simulink library "netZeroSpoolingController_ul"  (R2020a)
settings: Solver=VariableStepAuto  StartTime=0.0  StopTime=10.0  RelTol=1e-3
undefined symbols (not defined in the file or in its folder): fltCtrl, SPOOLINGCONTROLLER
libraries: simulink x8, runningAvg_ul x2, dspsigops x1, filteredPIDController_ul x1, stopwatch_ul x1
settings Model: Creator=James Reed  LastModifiedBy=Josh Gaming
settings DataIOCC: ReturnWorkspaceOutputs=off
settings DebuggingCC: ArithmeticOperatorsInVariantConditions=warning
settings SFSimCC: CustomCodeUndefinedFunction=UseInterfaceOnly

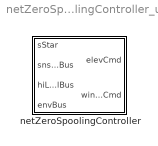
== system netZeroSpoolingController_ul ==
  netZeroSpoolingController : Subsystem  VariantControl=strcmpi(SPOOLINGCONTROLLER,'netZeroSpoolingController')  mask{reelInDefl=fltCtrl.elevatorReelInDef.Value, reelOutDefl=0, sigmaVecInit=[0.25 0.125], firstSpoolLap=fltCtrl.firstSpoolLap.Value}
      mask prompts: reelInDefl "Reel In Elevator Deflection [deg]"; reelOutDefl "Reel Out Elevator Deflection [deg]"; sigmaVecInit "Init Spooling Param Vec [center width]"; firstSpoolLap "First Lap to Begin Spooling"
      mask TypeOptions reelInDefl: ReelInElevDefl1/Value
      mask TypeOptions reelOutDefl: ReelOutElevDefl1/Value

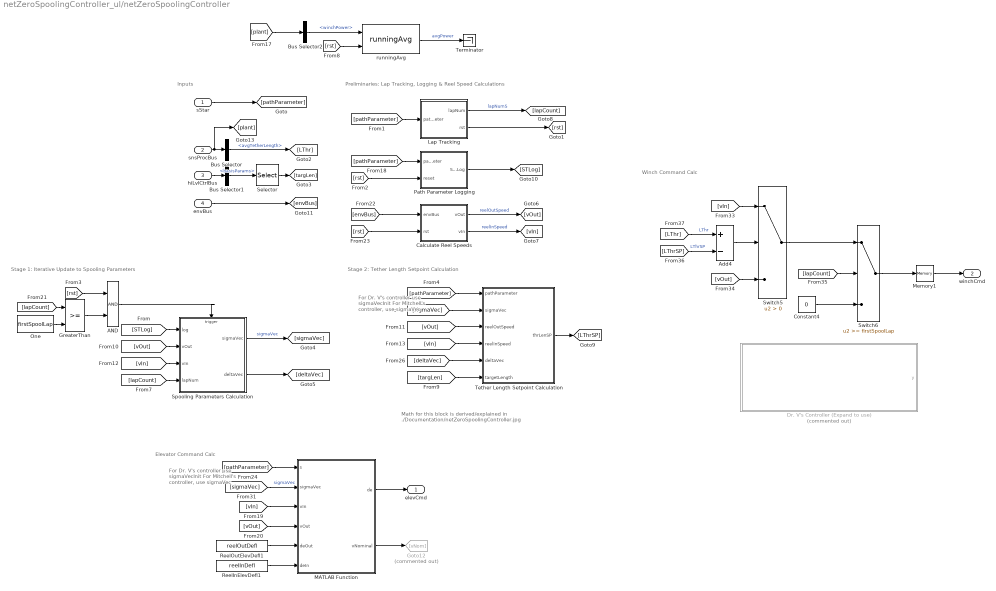
== system netZeroSpoolingController_ul/netZeroSpoolingController ==
  note: Elevator Command Calc
  note: Winch Command Calc
  note: For Dr. V's controller use sigmaVecInit
      |
      | For Mitchell's controller, use sigmaVec
  note: Math for this block is derived/explained in
      | ./Documentation/netZeroSpoolingController.jpg
  note: Stage 1: Iterative Update to Spooling Parameters
  note: Stage 2: Tether Length Setpoint Calculation
  note: Inputs
  note: Preliminaries: Lap Tracking, Logging & Reel Speed Calculations
  note: For Dr. V's controller use sigmaVecInit
      |
      | For Mitchell's controller, use sigmaVec
  "sStar " : Inport
  snsProcBus : Inport  Port=2  OutDataTypeStr=Bus: sensorsProcessingBus
  hiLvlCtrlBus : Inport  Port=3  OutDataTypeStr=Bus: hiLvlCtrlBus
  envBus : Inport  Port=4  OutDataTypeStr=Bus: envBus
  AND : Logic  AllPortsSameDT=off  OutDataTypeStr=boolean
  Add4 : Sum  Inputs=+-
  Bus Selector : BusSelector  OutputSignals=avgTetherLength
  Bus Selector1 : BusSelector  OutputSignals=basisParams
  Bus Selector2 : BusSelector  OutputSignals=winchPower
  Calculate Reel Speeds : Subsystem
  Constant4 : Constant  Value=0
  Dr. V's Controller (Expand to use) : Subsystem  Commented=on
  Goto12 : Goto  Commented=on  GotoTag=vNom
  GreaterThan : RelationalOperator  OutDataTypeStr=boolean  RndMeth=Simplest
  Lap Tracking : Subsystem
  MATLAB Function : MATLAB Function  TreatAsAtomicUnit=on
  Memory1 : Memory
  One : Constant  Value=firstSpoolLap  OutDataTypeStr=Inherit: Inherit via back propagation
  Path Parameter Logging : Subsystem
  ReelInElevDefl1 : Constant  Value=reelInDefl
  ReelOutElevDefl1 : Constant  Value=reelOutDefl
  Selector : Selector  InputPortWidth=5  IndexOptions=Index vector (dialog)  Indices=5  OutputSizes=1
  Spooling Parameters Calculation : Subsystem  TreatAsAtomicUnit=on
  Switch5 : Switch  Criteria=u2 > Threshold
  Switch6 : Switch  Threshold=firstSpoolLap
  Terminator : Terminator
  Tether Length Setpoint Calculation : Subsystem
  runningAvg : runningAvg_ul/runningAvg  SystemSampleTime=-1  Latency=0  AutoFrameSizeCalculation=off
  elevCmd : Outport  VectorParamsAs1DForOutWhenUnconnected=off
  "winchCmd " : Outport  Port=2  VectorParamsAs1DForOutWhenUnconnected=off
  wires:
  AND/1 -> Spooling Parameters Calculation/Trigger
  GreaterThan/1 -> AND/2
  [rst] -> AND/1
  One/1 -> GreaterThan/2
  [lapCount] -> GreaterThan/1
  hiLvlCtrlBus/1 -> Bus Selector1/1
  "sStar "/1 -> [pathParameter]
  Bus Selector/1 -> [LThr]  "<avgTetherLength>"
  Spooling Parameters Calculation/1(sigmaVec) -> [sigmaVec]  "sigmaVec"
  Spooling Parameters Calculation/2(deltaVec) -> [deltaVec]
  [vOut] -> Spooling Parameters Calculation/2(vOut)
  [vIn] -> Spooling Parameters Calculation/3(vIn)
  [pathParameter] -> Path Parameter Logging/1(pathParameter)
  [rst] -> Path Parameter Logging/2(reset)
  Path Parameter Logging/1(SVsTLog) -> [STLog]
  [STLog] -> Spooling Parameters Calculation/1(log)
  envBus/1 -> [envBus]
  [envBus] -> Calculate Reel Speeds/1(envBus)
  Calculate Reel Speeds/1(vOut) -> [vOut]  "reelOutSpeed"
  Calculate Reel Speeds/2(vIn) -> [vIn]  "reelInSpeed"
  [rst] -> Calculate Reel Speeds/2(rst)
  [pathParameter] -> Lap Tracking/1(pathParameter)
  Lap Tracking/1(lapNum) -> [lapCount]  "lapNumS"
  Lap Tracking/2(rst) -> [rst]
  [pathParameter] -> Tether Length Setpoint Calculation/1(pathParameter)
  [sigmaVec] -> Tether Length Setpoint Calculation/2(sigmaVec)
  [vOut] -> Tether Length Setpoint Calculation/3(reelOutSpeed)
  [vIn] -> Tether Length Setpoint Calculation/4(reelInSpeed)
  [deltaVec] -> Tether Length Setpoint Calculation/5(deltaVec)
  Tether Length Setpoint Calculation/1(thrLenSP) -> [LThrSP]
  [lapCount] -> Spooling Parameters Calculation/4(lapNum)
  Bus Selector1/1 -> Selector/1  "<basisParams>"
  Selector/1 -> [targLen]
  [targLen] -> Tether Length Setpoint Calculation/6(targetLength)
  [pathParameter] -> MATLAB Function/1(s)
  [vIn] -> MATLAB Function/3(vIn)
  [vOut] -> MATLAB Function/4(vOut)
  ReelInElevDefl1/1 -> MATLAB Function/6(deIn)
  ReelOutElevDefl1/1 -> MATLAB Function/5(deOut)
  MATLAB Function/1(de) -> elevCmd/1
  MATLAB Function/2(vNominal) -> Goto12/1
  [lapCount] -> Switch6/2
  Constant4/1 -> Switch6/3
  [LThrSP] -> Add4/2  "LThrSP"
  Add4/1 -> Switch5/2
  [vOut] -> Switch5/3
  Switch5/1 -> Switch6/1
  [vIn] -> Switch5/1
  [LThr] -> Add4/1  "LThr"
  [rst] -> runningAvg/2
  Bus Selector2/1 -> runningAvg/1  "<winchPower>"
  runningAvg/1 -> Terminator/1  "avgPower"
  snsProcBus/1 -> [plant], Bus Selector/1
  [plant] -> Bus Selector2/1
  [sigmaVec] -> MATLAB Function/2(sigmaVec)  "sigmaVec"
  Switch6/1 -> Memory1/1
  Memory1/1 -> "winchCmd "/1

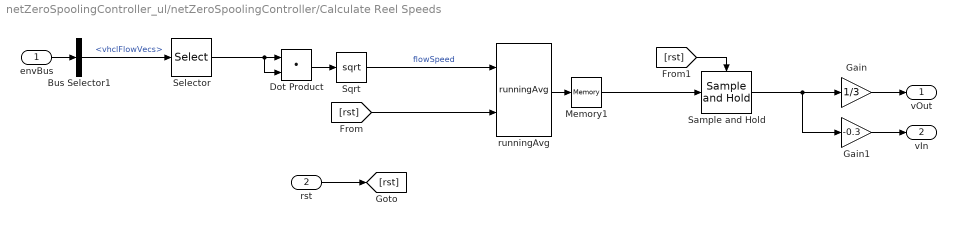
== system netZeroSpoolingController_ul/netZeroSpoolingController/Calculate Reel Speeds ==
  envBus : Inport
  rst : Inport  Port=2
  Bus Selector1 : BusSelector  OutputSignals=vhclFlowVecs
  Dot Product : DotProduct  InputSameDT=on  OutDataTypeStr=Inherit: Inherit via internal rule
  Gain : Gain  Gain=1/3
  Gain1 : Gain  Gain=-0.3
  Memory1 : Memory
  Sample and Hold : dspsigops/Sample and Hold  trig=Rising edge  initCond=0  latchinput=off
  Selector : Selector  NumberOfDimensions=2  InputPortWidth=3  IndexOptions=Select all,Index vector (dialog)  Indices=[1 3],5  OutputSizes=1,1
  Sqrt : Sqrt  SaturateOnIntegerOverflow=on
  runningAvg : runningAvg_ul/runningAvg  SystemSampleTime=-1  Latency=0  AutoFrameSizeCalculation=off
  vOut : Outport  VectorParamsAs1DForOutWhenUnconnected=off
  vIn : Outport  Port=2  VectorParamsAs1DForOutWhenUnconnected=off
  wires:
  Gain1/1 -> vIn/1
  Gain/1 -> vOut/1
  Sample and Hold/1 -> Gain1/1, Gain/1
  rst/1 -> [rst]
  Bus Selector1/1 -> Selector/1  "<vhclFlowVecs>"
  runningAvg/1 -> Memory1/1
  Sqrt/1 -> runningAvg/1  "flowSpeed"
  envBus/1 -> Bus Selector1/1
  Memory1/1 -> Sample and Hold/1
  [rst] -> runningAvg/2
  [rst] -> Sample and Hold/Trigger
  Selector/1 -> Dot Product/2, Dot Product/1
  Dot Product/1 -> Sqrt/1

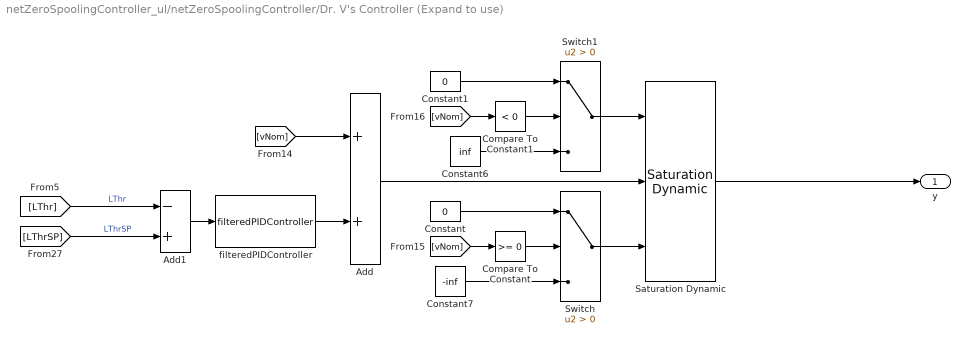
== system netZeroSpoolingController_ul/netZeroSpoolingController/Dr. V's Controller (Expand to use) ==
  Add : Sum
  Add1 : Sum  Inputs=-+
  Compare To Constant : simulink/Logic and Bit Operations/Compare To Constant  relop=>=  const=0  OutDataTypeStr=boolean
  Compare To Constant1 : simulink/Logic and Bit Operations/Compare To Constant  relop=<  const=0  OutDataTypeStr=boolean
  Constant : Constant  Value=0
  Constant1 : Constant  Value=0
  Constant6 : Constant  Value=inf
  Constant7 : Constant  Value=-inf
  Saturation Dynamic : simulink/Discontinuities/Saturation Dynamic  OutMin=[]  OutMax=[]  OutDataTypeStr=Inherit: Same as second input  OutDataType=fixdt(1, 16)  OutScaling=2^-10  DoSatur=off
  Switch : Switch  Criteria=u2 > Threshold
  Switch1 : Switch  Criteria=u2 > Threshold
  filteredPIDController : filteredPIDController_ul/filteredPIDController  kp=.1  ki=0  kd=0  Value=0  externalReset=none
  y : Outport
  wires:
  Compare To Constant1/1 -> Switch1/2
  Add/1 -> Saturation Dynamic/2
  [LThrSP] -> Add1/2  "LThrSP"
  [vNom] -> Compare To Constant/1
  Compare To Constant/1 -> Switch/2
  Add1/1 -> filteredPIDController/1
  Switch/1 -> Saturation Dynamic/3
  Constant6/1 -> Switch1/3
  filteredPIDController/1 -> Add/2
  Switch1/1 -> Saturation Dynamic/1
  [vNom] -> Compare To Constant1/1
  Constant/1 -> Switch/1
  [vNom] -> Add/1
  Constant1/1 -> Switch1/1
  [LThr] -> Add1/1  "LThr"
  Constant7/1 -> Switch/3
  Saturation Dynamic/1 -> y/1

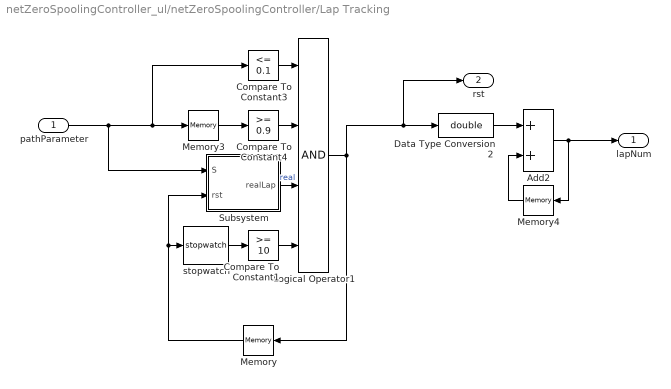
== system netZeroSpoolingController_ul/netZeroSpoolingController/Lap Tracking ==
  pathParameter : Inport
  Add2 : Sum
  Compare To Constant1 : simulink/Logic and Bit Operations/Compare To Constant  relop=>=  const=10  OutDataTypeStr=boolean
  Compare To Constant3 : simulink/Logic and Bit Operations/Compare To Constant  relop=<=  const=0.1  OutDataTypeStr=boolean
  Compare To Constant4 : simulink/Logic and Bit Operations/Compare To Constant  relop=>=  const=0.9  OutDataTypeStr=boolean
  Data Type Conversion2 : DataTypeConversion  OutDataTypeStr=double
  Logical Operator1 : Logic  Inputs=4  AllPortsSameDT=off  OutDataTypeStr=boolean
  Memory : Memory  InitialCondition=false
  Memory3 : Memory
  Memory4 : Memory
  Subsystem : Subsystem
  stopwatch : stopwatch_ul/stopwatch  SystemSampleTime=-1  Latency=0  AutoFrameSizeCalculation=off
  lapNum : Outport  VectorParamsAs1DForOutWhenUnconnected=off
  rst : Outport  Port=2  VectorParamsAs1DForOutWhenUnconnected=off
  wires:
  Compare To Constant3/1 -> Logical Operator1/1
  Memory3/1 -> Compare To Constant4/1
  Data Type Conversion2/1 -> Add2/1
  Logical Operator1/1 -> rst/1, Data Type Conversion2/1, Memory/1
  Memory4/1 -> Add2/2
  Add2/1 -> lapNum/1, Memory4/1
  Compare To Constant4/1 -> Logical Operator1/2
  pathParameter/1 -> Subsystem/1(S), Compare To Constant3/1, Memory3/1
  stopwatch/1 -> Compare To Constant1/1
  Memory/1 -> Subsystem/2(rst), stopwatch/1
  Compare To Constant1/1 -> Logical Operator1/4
  Subsystem/1(realLap) -> Logical Operator1/3  "real"

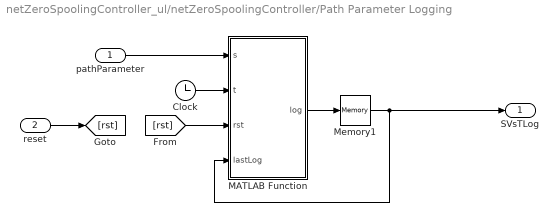
== system netZeroSpoolingController_ul/netZeroSpoolingController/Path Parameter Logging ==
  pathParameter : Inport
  reset : Inport  Port=2
  Clock : Clock
  MATLAB Function : MATLAB Function  TreatAsAtomicUnit=on
  Memory1 : Memory  InitialCondition=zeros(1000,2)
  SVsTLog : Outport  VectorParamsAs1DForOutWhenUnconnected=off
  wires:
  MATLAB Function/1(log) -> Memory1/1
  reset/1 -> [rst]
  pathParameter/1 -> MATLAB Function/1(s)
  Clock/1 -> MATLAB Function/2(t)
  Memory1/1 -> SVsTLog/1, MATLAB Function/4(lastLog)
  [rst] -> MATLAB Function/3(rst)

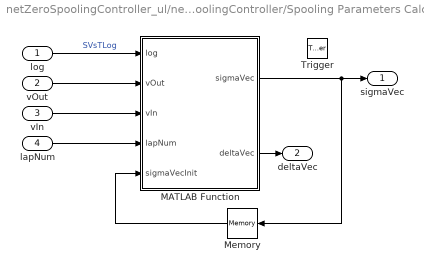
== system netZeroSpoolingController_ul/netZeroSpoolingController/Spooling Parameters Calculation ==
  log : Inport
  vOut : Inport  Port=2
  vIn : Inport  Port=3
  lapNum : Inport  Port=4
  Trigger : TriggerPort  VariantControl=Variant
  MATLAB Function : MATLAB Function  TreatAsAtomicUnit=on
  Memory : Memory  InitialCondition=sigmaVecInit  InheritSampleTime=on
  sigmaVec : Outport  InitialOutput=sigmaVecInit  VectorParamsAs1DForOutWhenUnconnected=off
  deltaVec : Outport  Port=2  InitialOutput="[0.0136    0.0097    0.0198    0.0152    0.0208]"  VectorParamsAs1DForOutWhenUnconnected=off
  wires:
  log/1 -> MATLAB Function/1(log)  "SVsTLog"
  Memory/1 -> MATLAB Function/5(sigmaVecInit)
  vOut/1 -> MATLAB Function/2(vOut)
  vIn/1 -> MATLAB Function/3(vIn)
  MATLAB Function/2(deltaVec) -> deltaVec/1
  MATLAB Function/1(sigmaVec) -> Memory/1, sigmaVec/1
  lapNum/1 -> MATLAB Function/4(lapNum)

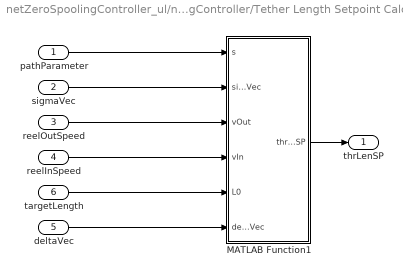
== system netZeroSpoolingController_ul/netZeroSpoolingController/Tether Length Setpoint Calculation ==
  pathParameter : Inport
  sigmaVec : Inport  Port=2
  reelOutSpeed : Inport  Port=3
  reelInSpeed : Inport  Port=4
  deltaVec : Inport  Port=5
  targetLength : Inport  Port=6
  MATLAB Function1 : MATLAB Function  TreatAsAtomicUnit=on
  thrLenSP : Outport  VectorParamsAs1DForOutWhenUnconnected=off
  wires:
  sigmaVec/1 -> MATLAB Function1/2(sigmaVec)
  reelInSpeed/1 -> MATLAB Function1/4(vIn)
  reelOutSpeed/1 -> MATLAB Function1/3(vOut)
  pathParameter/1 -> MATLAB Function1/1(s)
  MATLAB Function1/1(thrLenSP) -> thrLenSP/1
  deltaVec/1 -> MATLAB Function1/6(deltaVec)
  targetLength/1 -> MATLAB Function1/5(L0)

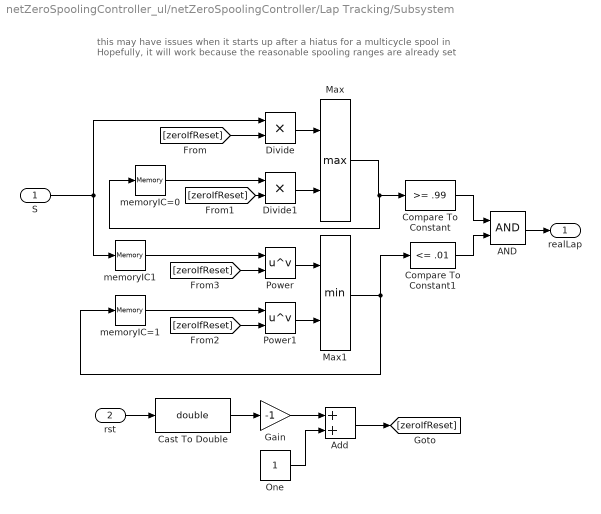
== system netZeroSpoolingController_ul/netZeroSpoolingController/Lap Tracking/Subsystem ==
  note: this may have issues when it starts up after a hiatus for a multicycle spool in
      | Hopefully, it will work because the reasonable spooling ranges are already set
  S : Inport
  rst : Inport  Port=2
  AND : Logic  AllPortsSameDT=off  OutDataTypeStr=boolean
  Add : Sum
  Cast To Double : DataTypeConversion  OutDataTypeStr=double
  Compare To Constant : simulink/Logic and Bit Operations/Compare To Constant  relop=>=  const=.99  OutDataTypeStr=boolean
  Compare To Constant1 : simulink/Logic and Bit Operations/Compare To Constant  relop=<=  const=.01  OutDataTypeStr=boolean
  Divide : Product  Inputs=**
  Divide1 : Product  Inputs=**
  Gain : Gain  Gain=-1
  Max : MinMax  Function=max  Inputs=2
  Max1 : MinMax  Inputs=2
  One : Constant  OutDataTypeStr=Inherit: Inherit via back propagation
  Power : Math  Operator=pow  SaturateOnIntegerOverflow=on
  Power1 : Math  Operator=pow  SaturateOnIntegerOverflow=on
  memoryIC1 : Memory  InitialCondition=1
  memoryIC=0 : Memory
  memoryIC=1 : Memory  InitialCondition=1
  realLap : Outport
  wires:
  Max1/1 -> Compare To Constant1/1, memoryIC=1/1
  rst/1 -> Cast To Double/1
  S/1 -> Divide/1, memoryIC1/1
  Gain/1 -> Add/1
  Add/1 -> [zeroIfReset]
  One/1 -> Add/2
  Divide/1 -> Max/1
  Max/1 -> memoryIC=0/1, Compare To Constant/1
  Power/1 -> Max1/1
  Power1/1 -> Max1/2
  Cast To Double/1 -> Gain/1
  Compare To Constant/1 -> AND/1
  Compare To Constant1/1 -> AND/2
  AND/1 -> realLap/1
  [zeroIfReset] -> Divide/2
  [zeroIfReset] -> Power/2
  [zeroIfReset] -> Divide1/2
  Divide1/1 -> Max/2
  memoryIC=0/1 -> Divide1/1
  [zeroIfReset] -> Power1/2
  memoryIC=1/1 -> Power1/1
  memoryIC1/1 -> Power/1

== matlab function netZeroSpoolingController_ul/netZeroSpoolingController/Spooling Parameters Calculation/MATLAB Function ==
  data: log input; vOut input; vIn input; lapNum input; sigmaVecInit input; sigmaVec output; deltaVec output
function [sigmaVec,deltaVec] = fcn(log,vOut,vIn,lapNum,sigmaVecInit)

sc = sigmaVecInit(1);
sw = sigmaVecInit(2);
sigmaVec = sigmaVecInit;

cleanLog = [0 0;...
    log(and(log(:,1)~=0,log(:,2)~=0),:)];
 
% Extract regions
r1 = cleanLog(and(cleanLog(:,1)>=0        ,cleanLog(:,1)<sc-sw),:);
r2 = cleanLog(and(cleanLog(:,1)>=sc-sw    ,cleanLog(:,1)<sc+sw),:);
r3 = cleanLog(and(cleanLog(:,1)>=sc+sw    ,cleanLog(:,1)<0.5+sc-sw),:);
r4 = cleanLog(and(cleanLog(:,1)>=0.5+sc-sw,cleanLog(:,1)<0.5+sc+sw),:);
r5 = cleanLog(and(cleanLog(:,1)>=0.5+sc+sw,cleanLog(:,1)<=1),:);

% Calculate average numerical derivative in each region ds/dt
ds1 = mean(diff(r1(:,1))./diff(r1(:,2)));
ds2 = mean(diff(r2(:,1))./diff(r2(:,2)));
ds3 = mean(diff(r3(:,1))./diff(r3(:,2)));
ds4 = mean(diff(r4(:,1))./diff(r4(:,2)));
ds5 = mean(diff(r5(:,1))./diff(r5(:,2)));

deltaVec = [ds1 ds2 ds3 ds4 ds5]';

dsInv = diag([1/ds1 1/ds2 1/ds3 1/ds4 1/ds5]);

V = diag([vOut vIn vOut vIn vOut]);

Delta = eye(5);
Delta(2,1) = -1;
Delta(3,2) = -1;
Delta(4,3) = -1;
Delta(5,4) = -1;

A  = [ 0  0 0.5 0.5 1]';
B1 = [ 1  1   1   1 0]';
B2 = [-1  1  -1   1 0]';

c1 = ones(1,5)*V*dsInv*Delta*(A+B1*sc);
c2 = ones(1,5)*V*dsInv*Delta*B2;
sw = min([max([-c1/c2 0]) sc]); % 0<=sw<=sc
sigmaVec(2) = sw;

% Note: the following code alternates between updating sc and sw.
% After a bit of testing, I found that the update on sc was really screwing
% things up.  Not sure why that is at the moment, but it's kind of
% irrelevant since the update on sw alone works well enough.  Moving on.
% -MC

% Alternate updaing sc and sw each lap
% if mod(round(lapNum),2) % Odd lap number
    % Case 1, sc fixed, update sw
%     sigmaVec(1) = sc;
%     c1 = ones(1,5)*V*dsInv*Delta*(A+B1*sc);
%     c2 = ones(1,5)*V*dsInv*Delta*B2;
%     sw = min([max([-c1/c2 0]) sc]); % 0<=sw<=0.25
% else % Even lap number
%     % Case 2, sw fixed, update sc
% %     sigmaVec(2) = sw;
%     c1 = ones(1,5)*V*dsInv*Delta*(A+B2*sw);
%     c2 = ones(1,5)*V*dsInv*Delta*B1;
%     sc = min([max([-c1/c2 sw]) 0.5-sw]);
% end

% sigmaVec(1) = sc;
% sigmaVec(2) = sw;

== matlab function netZeroSpoolingController_ul/netZeroSpoolingController/Path Parameter Logging/MATLAB Function ==
  data: s input; log output; t input; rst input; lastLog input
function log = fcn(s,t,rst,lastLog)
% function that logs the path position and time into a matrix
% [pathPosition,t]
if rst
    lastLog = nan(1000,2);
end
log = lastLog;
idx = min([max([round(s*1000),1]),1000]);
log(idx,1) = s;
log(idx,2) = t;

== matlab function netZeroSpoolingController_ul/netZeroSpoolingController/Tether Length Setpoint Calculation/MATLAB Function1 ==
  data: s input; thrLenSP output; sigmaVec input; vOut input; vIn input; L0 input; deltaVec input
function thrLenSP  = fcn(s,sigmaVec,vOut,vIn,L0,deltaVec)

thrLenSP = LThrInt(s,sigmaVec,vOut,vIn,L0,deltaVec);

end

== matlab function netZeroSpoolingController_ul/netZeroSpoolingController/MATLAB Function ==
  data: de output; s input; vNominal output; sigmaVec input; vIn input; vOut input; deOut input; deIn input
function [de,vNominal] = fcn(s,sigmaVec,vIn,vOut,deOut,deIn)
vNominal = vOut;
de = deOut;

sc = sigmaVec(1);
sw = sigmaVec(2);

if s>=sc-sw && s<=sc+sw
    vNominal = vIn;
    de = deIn;
    return
end

if s>=0.5+sc-sw && s<=0.5+sc+sw
    vNominal = vIn;
    de = deIn;
    return
end
end
